simulink model "particle_model"  (R2021a)
settings: Solver=FixedStepAuto  StartTime=0.0  StopTime=10  FixedStep=0.05  RelTol=1e-3
values from neighbouring files (symbols this model uses):
  Iz = 1    [particle_mpc.m]
  m = length(arch_type)    [batch_simulation.m]    (also in particle_mpc.m = 1)
  sys_d = c2d(sys, ts)    [particle_mpc.m]
  ts = 0.05    [particle_mpc.m]
libraries: nesl_utility x8, mpclib x1
settings Model: Creator=victor  LastModifiedBy=victor

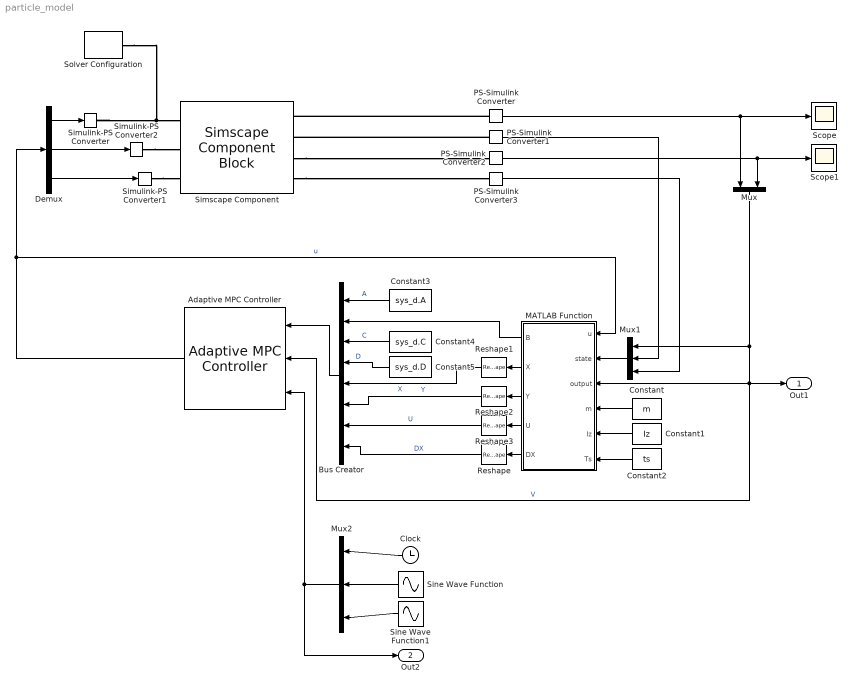
== system particle_model ==
  Adaptive MPC Controller : mpclib/Adaptive MPC Controller  SCDEnableBlockLinearizationSpecification=on  mpcobj=mpc_controller  enable_value=0  updateMPCinCallerWorkspace=on  md_inport=off  mv_inport=off  uref_inport=off  return_cost=off  return_mvseq=off  return_qpstatus=off  return_xseq=off  return_state=off  return_ovseq=off  state_inport=off  isltv_plant=off  umin_inport=off  umax_inport=off  ymin_inport=off  ymax_inport=off  cc_inport=off  ywt_inport=off  uwt_inport=off  duwt_inport=off  rhoeps_inport=off  pm_inport=off  MaximumP=10  HorizonChoice=FixedHorizon  BlockDataType=double  SampleTimeInherited=off  switch_inport=off
  Bus Creator : BusCreator  Inputs=8
  Clock : Clock
  Constant : Constant  Value=m
  Constant1 : Constant  Value=Iz
  Constant2 : Constant  Value=ts
  Constant3 : Constant  Value=sys_d.A
  Constant4 : Constant  Value=sys_d.C
  Constant5 : Constant  Value=sys_d.D
  Demux : Demux  Outputs=3
  MATLAB Function : MATLAB Function  TreatAsAtomicUnit=on
  Mux : Mux  Inputs=2
  Mux1 : Mux  Inputs=3
  Mux2 : Mux  Inputs=3
  PS-Simulink Converter{,1..3} (4 alike) : nesl_utility/PS-Simulink Converter  PhysicalDomain=network_engine_domain  SubClassName=ps_output  LeftPortType=input  RightPortType=output  PseudoPeriodic=off  Frequencies=[]  Unit=inherit  AffineConversion=off
      settings: SourceProductBaseCode=PW,SS
  Reshape : Reshape  OutputDimensionality=Customize  OutputDimensions=[6, 1]
  Reshape1 : Reshape  OutputDimensionality=Customize  OutputDimensions=[6, 1]
  Reshape2 : Reshape  OutputDimensionality=Customize  OutputDimensions=[3, 1]
  Reshape3 : Reshape  OutputDimensionality=Customize  OutputDimensions=[3, 1]
  Scope : Scope
  Scope1 : Scope
  Simscape Component : SimscapeComponentBlock  SourceFile=particle  ComponentPath=particle  ComponentVariants="[\"particle\"]"  ComponentVariantNames="[\"particle\"]"  ClassName=particle  SchemaVersion=1  mass=1 kg  Iz=1 kg*m^2  x_specify=off  x_priority=None  x=0 m  x_nominal_specify=off  x_nominal_unit=m  x_nominal_value=1  dx_specify=off  dx_priority=None  dx=0 m/s  dx_nominal_specify=off  dx_nominal_unit=m/s  dx_nominal_value=1  y_specify=off  y_priority=None  y=0 m  y_nominal_specify=off  y_nominal_unit=m  y_nominal_value=1  dy_specify=off  dy_priority=None  dy=0 m/s  dy_nominal_specify=off  dy_nominal_unit=m/s  dy_nominal_value=1  theta_specify=off  theta_priority=None  theta=0 rad  theta_nominal_specify=off  theta_nominal_unit=rad  theta_nominal_value=1  dtheta_specify=off  dtheta_priority=None  dtheta=0 rad/s  dtheta_nominal_specify=off  dtheta_nominal_unit=rad/s  dtheta_nominal_value=1
      settings: CopyFcn=simscape.engine.sli.internal.componentblockcallback(gcbh,'COPY')  PreCopyFcn=simscape.engine.sli.internal.componentblockcallback(gcbh,'PRECOPY')  PreDeleteFcn=simscape.engine.sli.internal.componentblockcallback(gcbh,'PREDELETE')  InternalSimscapePortConfiguration="{\"Bottom\":[],\"Left\":[{\"id\":\"fx\",\"label\":\"fx\",\"type\":\"input\"},{\"id\":\"fy\",\"label\":\"fy\",\"type\":\"input\"},{\"id\":\"Mz\",\"label\":\"Mz\",\"type\":\"input\"}],\"Right\":[{\"id\":\"pos\",\"label\":\"pos\",\"type\":\"output\"},{\"id\":\"velocity\",\"label\":\"velocity\",\"type\":\"output\"},{\"id\":\"angle\",\"label\":\"angle\",\"type\":\"output\"},{\"id\":\"angular_vel\",\"label\":\"angular_vel\",\"type\":\"output\"}],\"Top\":[]}"
      mask Type: particle
  Simulink-PS Converter : nesl_utility/Simulink-PS Converter  PhysicalDomain=network_engine_domain  SubClassName=ps_input  LeftPortType=input  RightPortType=output  PseudoPeriodic=off  Frequencies=[]  NoiseDistribution=none  NoiseParameters=[]  Unit=1  AffineConversion=off  FilteringAndDerivatives=provide  SimscapeFilterOrder=1  InputFilterTimeConstant=0.001  UdotUserProvided=0
      settings: SourceProductBaseCode=PW,SS
  Simulink-PS Converter1 : nesl_utility/Simulink-PS Converter  PhysicalDomain=network_engine_domain  SubClassName=ps_input  LeftPortType=input  RightPortType=output  PseudoPeriodic=off  Frequencies=[]  NoiseDistribution=none  NoiseParameters=[]  Unit=1  AffineConversion=off  FilteringAndDerivatives=provide  SimscapeFilterOrder=1  InputFilterTimeConstant=0.001  UdotUserProvided=0
      settings: SourceProductBaseCode=PW,SS
  Simulink-PS Converter2 : nesl_utility/Simulink-PS Converter  PhysicalDomain=network_engine_domain  SubClassName=ps_input  LeftPortType=input  RightPortType=output  PseudoPeriodic=off  Frequencies=[]  NoiseDistribution=none  NoiseParameters=[]  Unit=1  AffineConversion=off  FilteringAndDerivatives=provide  SimscapeFilterOrder=1  InputFilterTimeConstant=0.001  UdotUserProvided=0
      settings: SourceProductBaseCode=PW,SS
  Sine Wave Function : Sin  SampleTime=0
  Sine Wave Function1 : Sin  Phase=pi/2  SampleTime=0
  Solver Configuration : nesl_utility/Solver Configuration  PhysicalDomain=network_engine_domain  SubClassName=solver  LeftPortType=input  RightPortType=generic  Tones=[]  Harmonics=[]  SimulateNoise=off  Profile=off  UseLocalSampling=off  EnableSwitchedLinearOptims=on  FrequencyDomain=off  UseCCode=off  RelTol=0.001  AbsTol=1e-06  MinStep=1e-09  ToWorkspace=off  RevertToSquareIcSolve=off  NumHomotopyIterations=100  PhasorMode=off  PhasorModeNumHarmonics=1  DoDC=off  ResidualTolerance=1e-09  UseLocalSolver=off  LocalSolverChoice=NE_BACKWARD_EULER_ADVANCER  LocalSolverSampleTime=0.001  DoFixedCost=off  MaxNonlinIter=3  MaxModeIter=2  ComputeImpulses=off  ImpulseIterations=2  LinearAlgebra=auto  EquationFormulation=NE_TIME_EF  DelaysMemoryBudget=1024  AutomaticFiltering=on  FilteringTimeConstant=0.001  PartitionStorageMethod=AS_NEEDED  PartitionMemoryBudget=1024  PartitionMethod=ROBUST
      settings: SourceProductBaseCode=PW,SS
  Out1 : Outport  SignalName=model_output
  Out2 : Outport  Port=2  SignalName=model_output
  wires:
  PS-Simulink Converter/1 -> Mux/1, Scope/1
  Demux/3 -> Simulink-PS Converter1/1
  Mux/1 -> Mux1/1, MATLAB Function/3(output), Adaptive MPC Controller/2, Out1/1  "V"
  Demux/1 -> Simulink-PS Converter/1
  Demux/2 -> Simulink-PS Converter2/1
  Adaptive MPC Controller/1 -> MATLAB Function/1(u), Demux/1  "u"
  MATLAB Function/1(B) -> Bus Creator/2
  MATLAB Function/2(X) -> Reshape1/1
  Bus Creator/1 -> Adaptive MPC Controller/1
  PS-Simulink Converter2/1 -> Mux/2, Scope1/1
  Mux1/1 -> MATLAB Function/2(state)
  PS-Simulink Converter1/1 -> Mux1/2
  PS-Simulink Converter3/1 -> Mux1/3
  Constant/1 -> MATLAB Function/4(m)
  Constant1/1 -> MATLAB Function/5(Iz)
  Constant2/1 -> MATLAB Function/6(Ts)
  Constant3/1 -> Bus Creator/1  "A"
  Constant4/1 -> Bus Creator/3  "C"
  Constant5/1 -> Bus Creator/4  "D"
  MATLAB Function/5(DX) -> Reshape/1
  Reshape/1 -> Bus Creator/8  "DX"
  Reshape1/1 -> Bus Creator/5  "X"
  MATLAB Function/3(Y) -> Reshape2/1
  Reshape2/1 -> Bus Creator/6  "Y"
  MATLAB Function/4(U) -> Reshape3/1
  Reshape3/1 -> Bus Creator/7  "U"
  Mux2/1 -> Adaptive MPC Controller/3, Out2/1
  Sine Wave Function1/1 -> Mux2/3
  Clock/1 -> Mux2/1
  Sine Wave Function/1 -> Mux2/2
  connections:
  PS-Simulink Converter/LConn1 -- Simscape Component/RConn1
  Simulink-PS Converter/RConn1 -- Simscape Component/LConn1 -- Solver Configuration/RConn1
  PS-Simulink Converter1/LConn1 -- Simscape Component/RConn2
  Simulink-PS Converter1/RConn1 -- Simscape Component/LConn3
  Simulink-PS Converter2/RConn1 -- Simscape Component/LConn2
  Simscape Component/RConn3 -- PS-Simulink Converter2/LConn1
  Simscape Component/RConn4 -- PS-Simulink Converter3/LConn1

== matlab function particle_model/MATLAB Function ==
  data: u input; state input; output input; B output; X output; Y output; U output; DX output; m input; Iz input; Ts input
function [B, X, Y, U, DX] = fcn(u, state, output, m, Iz, Ts)
    A_c = [0 0 0 1 0 0;
     0 0 0 0 1 0;
     0 0 0 0 0 1;
     0 0 0 0 0 0;
     0 0 0 0 0 0;
     0 0 0 0 0 0];
    B = [zeros(3,3); 
          [cos(output(3))/m -sin(output(3))/m 0;
           sin(output(3))/m  cos(output(3))/m 0;
           0          0         1/Iz]];

    B = B*Ts; % zero order hold discretization
    X = state;
    Y = output;
    U = u;
    DX = A_c*Ts*state + B*U;
    DX = reshape(DX, [6 1]);
end
